simulink model "Simulink_4"  (Simulink 10.0)
settings: Solver=ode45  StartTime=0.0  StopTime=100.0  RelTol=1e-5  EnableMultiTasking=on
libraries: simulink x1
settings Model: Creator=unknown  LastModifiedBy=unknown
settings DataIOCC: LimitDataPoints=on  SignalLoggingSaveFormat=ModelDataLogs  SignalLoggingName=sigsOut
settings OptimizationCC: LifeSpan=auto
settings DebuggingCC: SaveWithParameterizedLinksMsg=none  SignalResolutionControl=TryResolveAllWithWarning  MultiTaskDSMMsg=warning  MultiTaskCondExecSysMsg=none  SFUnexpectedBacktrackingDiag=error  SFNoUnconditionalDefaultTransitionDiag=error  SFExecutionAtInitializationDiag=warning  ArithmeticOperatorsInVariantConditions=error
settings HardwareCC: TargetUnknown=on
settings SFSimCC: SimUseLocalCustomCode=on  CustomCodeUndefinedFunction=FilterOut
settings RTWCC: RTWUseLocalCustomCode=on
settings CodeAppCC: StateflowObjectComments=off
settings GRTTargetCC: TargetLangStandard=C99 (ISO)

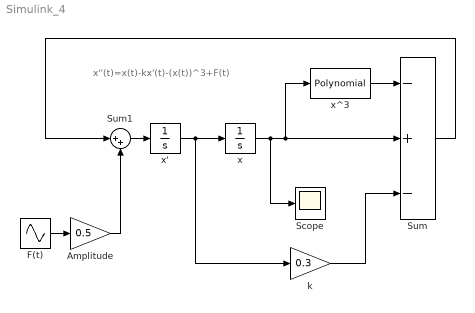
== system Simulink_4 ==
  note: x''(t)=x(t)-kx'(t)-(x(t))^3+F(t)
  Amplitude : Gain  Gain=0.5  SaturateOnIntegerOverflow=on  OutDataTypeStr=Inherit: Same as input  ParamDataTypeStr=Inherit: Same as input
  F(t) : Sin  Frequency=1.25  Phase=pi/2  SampleTime=0
  Scope : Scope
  Sum : Sum  Inputs=-+-  SaturateOnIntegerOverflow=on
  Sum1 : Sum  Inputs=|++  SaturateOnIntegerOverflow=on
  k : Gain  Gain=0.3  SaturateOnIntegerOverflow=on  OutDataTypeStr=Inherit: Same as input  ParamDataTypeStr=Inherit: Same as input
  x : Integrator  InitialCondition=1
  x' : Integrator  InitialCondition=1
  x^3 : simulink/Math Operations/Polynomial  coefs=[1,0,0,0]
      settings: SourceProductName=Simulink  SourceProductBaseCode=SL
  wires:
  x'/1 -> x/1, k/1
  x/1 -> Scope/1, Sum/2, x^3/1
  Sum1/1 -> x'/1
  k/1 -> Sum/3
  Sum/1 -> Sum1/1
  x^3/1 -> Sum/1
  F(t)/1 -> Amplitude/1
  Amplitude/1 -> Sum1/2
